simulink model "untitled"  (R2022b)
settings: Solver=FixedStepDiscrete  StartTime=0.0  StopTime=10.0  FixedStep=1e-3  RelTol=1e-3  EnableMultiTasking=on
libraries: arduinolib x4
settings Model: ExtModeTrigDuration=2  Creator=yasso  LastModifiedBy=yasso
settings OptimizationCC: EnhancedBackFolding=on  PassReuseOutputArgsAs=Individual arguments  ZeroExternalMemoryAtStartup=off  ZeroInternalMemoryAtStartup=off  MaxStackSize=64  OptimizeBlockOrder=speed  DifferentSizesBufferReuse=on  OptimizationCustomize=off  EfficientTunableParamExpr=on
settings DebuggingCC: ParameterTunabilityLossMsg=error
settings HardwareCC: ProdBitPerInt=16  ProdBitPerPointer=16  ProdBitPerSizeT=16  ProdBitPerPtrDiffT=16  ProdLargestAtomicFloat=None  ProdWordSize=8  ProdHWDeviceType=Atmel->AVR
settings SFSimCC: MATLABDynamicMemAlloc=off
settings RTWCC: Description=Embedded Coder  SystemTargetFile=ert.tlc  HardwareBoard=Arduino Uno  TLCOptions=-aInlineSetEventsForThisBaseRateFcn=TLC_FALSE -aSuppressMultiTaskScheduler=TLC_FALSE -aRateBasedStepFcn=1  TemplateMakefile=ert_default_tmf  Toolchain=Arduino AVR  BuildConfiguration=Faster Runs
settings CodeAppCC: ForceParamTrailComments=on  IgnoreCustomStorageClasses=off  OperatorAnnotations=on  SimulinkDataObjDesc=on  SFDataObjDesc=on  InsertBlockDesc=on
settings ERTTargetCC: SupportContinuousTime=on  SupportVariableSizeSignals=on  ExtModeTransport=3  ExtModeStaticAlloc=on  ExtModeAutomaticAllocSize=off  ExtModeStaticAllocSize=250  ExtModeMexFile=ext_xcp  ExtModeIntrfLevel=Level2 - Open

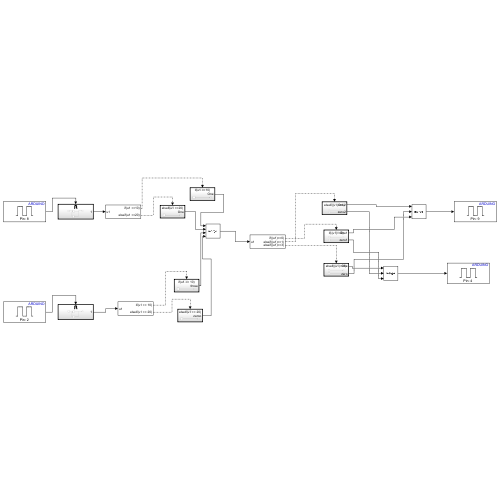
[thumbnail: Simulink's stored preview of the top-level diagram]
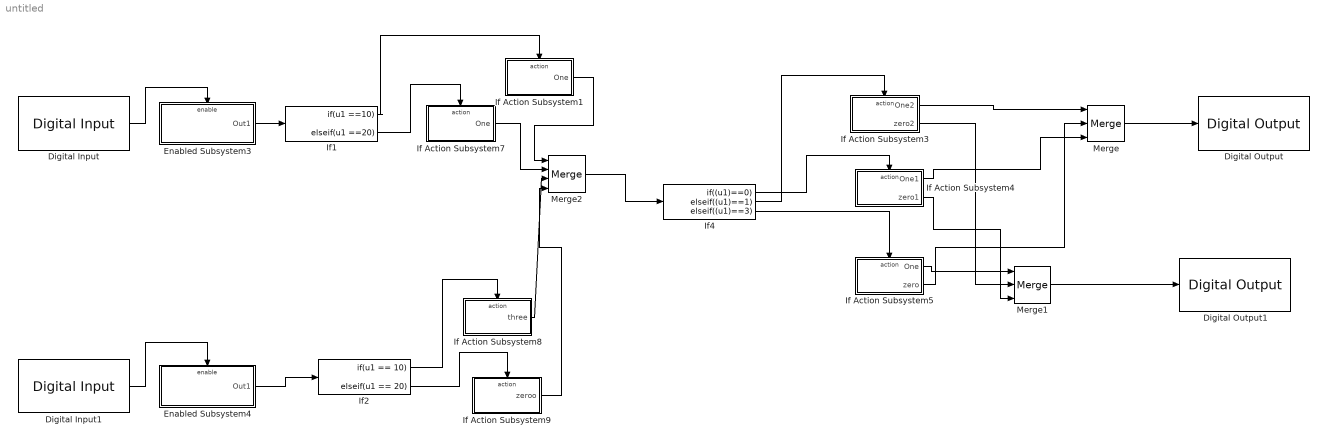
== system untitled ==
  Digital Input : arduinolib/Digital Input  pinNumber=8  mode=Default  Direction=input  SampleTime=0.1  blockPlatform=arduino
  Digital Input1 : arduinolib/Digital Input  pinNumber=2  mode=Default  Direction=input  SampleTime=0.1  blockPlatform=arduino
  Digital Output : arduinolib/Digital Output  pinNumber=9  Direction=output  blockPlatform=arduino
  Digital Output1 : arduinolib/Digital Output  pinNumber=4  Direction=output  blockPlatform=arduino
  Enabled Subsystem3 : Subsystem  TreatAsAtomicUnit=on
  Enabled Subsystem4 : Subsystem  TreatAsAtomicUnit=on
  If Action Subsystem1 : Subsystem  TreatAsAtomicUnit=on
  If Action Subsystem3 : Subsystem  TreatAsAtomicUnit=on
  If Action Subsystem4 : Subsystem  TreatAsAtomicUnit=on
  If Action Subsystem5 : Subsystem  TreatAsAtomicUnit=on
  If Action Subsystem7 : Subsystem  TreatAsAtomicUnit=on
  If Action Subsystem8 : Subsystem  TreatAsAtomicUnit=on
  If Action Subsystem9 : Subsystem  TreatAsAtomicUnit=on
  If1 : If  IfExpression=u1 ==10  ElseIfExpressions=u1 ==20  ShowElse=off
  If2 : If  IfExpression=u1 == 10  ElseIfExpressions=u1 == 20  ShowElse=off
  If4 : If  IfExpression=(u1)==0  ElseIfExpressions=(u1)==1,(u1)==3  ShowElse=off
  Merge : Merge  Inputs=3
  Merge1 : Merge  Inputs=3
  Merge2 : Merge  Inputs=4
  wires:
  If Action Subsystem8/1(three) -> Merge2/3
  If Action Subsystem9/1(zeroo) -> Merge2/4
  If2/1 -> If Action Subsystem8/Action
  If Action Subsystem4/1(One1) -> Merge/3
  If Action Subsystem5/1(One) -> Merge1/1
  Digital Input/1 -> Enabled Subsystem3/Enable
  If Action Subsystem1/1(One) -> Merge2/1
  Merge2/1 -> If4/1
  If1/2 -> If Action Subsystem7/Action
  Enabled Subsystem4/1(Out1) -> If2/1
  If1/1 -> If Action Subsystem1/Action
  Enabled Subsystem3/1(Out1) -> If1/1
  If2/2 -> If Action Subsystem9/Action
  If Action Subsystem4/2(zero1) -> Merge1/3
  If Action Subsystem7/1(One) -> Merge2/2
  Merge1/1 -> Digital Output1/1
  Merge/1 -> Digital Output/1
  If4/1 -> If Action Subsystem4/Action
  Digital Input1/1 -> Enabled Subsystem4/Enable
  If Action Subsystem3/2(zero2) -> Merge1/2
  If Action Subsystem3/1(One2) -> Merge/1
  If Action Subsystem5/2(zero) -> Merge/2
  If4/3 -> If Action Subsystem5/Action
  If4/2 -> If Action Subsystem3/Action

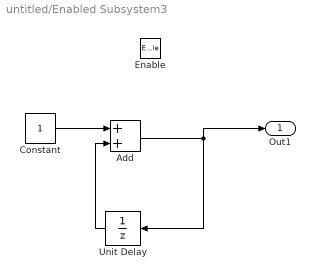
== system untitled/Enabled Subsystem3 ==
  Enable : EnablePort  StatesWhenEnabling=reset
  Add : Sum
  Constant : Constant
  Unit Delay : UnitDelay  SampleTime=-1  HasFrameUpgradeWarning=on
  Out1 : Outport
  wires:
  Unit Delay/1 -> Add/2
  Add/1 -> Out1/1, Unit Delay/1
  Constant/1 -> Add/1

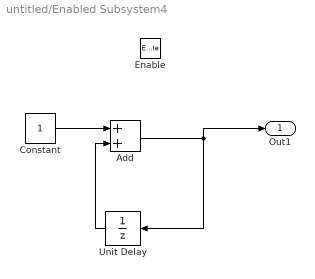
== system untitled/Enabled Subsystem4 ==
  Enable : EnablePort  StatesWhenEnabling=reset
  Add : Sum
  Constant : Constant
  Unit Delay : UnitDelay  SampleTime=-1  HasFrameUpgradeWarning=on
  Out1 : Outport
  wires:
  Constant/1 -> Add/1
  Add/1 -> Unit Delay/1, Out1/1
  Unit Delay/1 -> Add/2

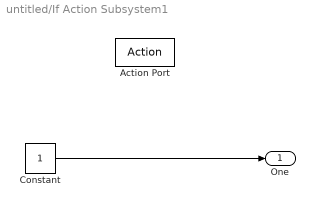
== system untitled/If Action Subsystem1 ==
  Action Port : ActionPort  ActionPortLabel=if(u1 ==10)
  Constant : Constant
  One : Outport
  wires:
  Constant/1 -> One/1

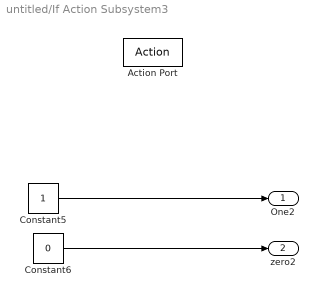
== system untitled/If Action Subsystem3 ==
  Action Port : ActionPort  ActionPortLabel=elseif((u1)==1)
  Constant5 : Constant
  Constant6 : Constant  Value=0
  One2 : Outport
  zero2 : Outport  Port=2
  wires:
  Constant5/1 -> One2/1
  Constant6/1 -> zero2/1

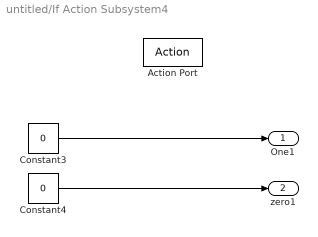
== system untitled/If Action Subsystem4 ==
  Action Port : ActionPort  ActionPortLabel=if((u1)==0)
  Constant3 : Constant  Value=0
  Constant4 : Constant  Value=0
  One1 : Outport
  zero1 : Outport  Port=2
  wires:
  Constant4/1 -> zero1/1
  Constant3/1 -> One1/1

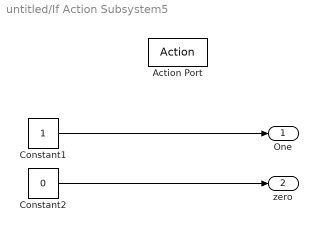
== system untitled/If Action Subsystem5 ==
  Action Port : ActionPort  ActionPortLabel=elseif((u1)==3)
  Constant1 : Constant
  Constant2 : Constant  Value=0
  One : Outport
  zero : Outport  Port=2
  wires:
  Constant1/1 -> One/1
  Constant2/1 -> zero/1

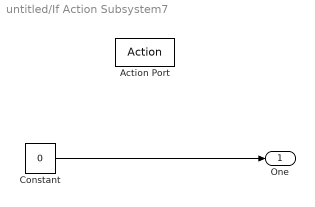
== system untitled/If Action Subsystem7 ==
  Action Port : ActionPort  ActionPortLabel=elseif(u1 ==20)
  Constant : Constant  Value=0
  One : Outport
  wires:
  Constant/1 -> One/1

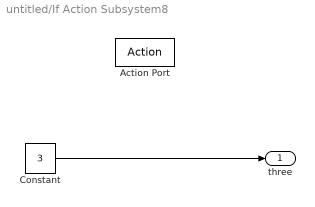
== system untitled/If Action Subsystem8 ==
  Action Port : ActionPort  ActionPortLabel=if(u1 == 10)
  Constant : Constant  Value=3
  three : Outport
  wires:
  Constant/1 -> three/1

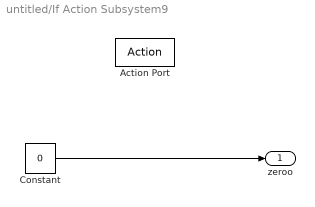
== system untitled/If Action Subsystem9 ==
  Action Port : ActionPort  ActionPortLabel=elseif(u1 == 20)
  Constant : Constant  Value=0
  zeroo : Outport
  wires:
  Constant/1 -> zeroo/1
